simulink model "D53_LKAS_JLU_20200903_0931"  (R2018b)
settings: Solver=ode3  StartTime=0.0  StopTime=10.0  FixedStep=0.01  RelTol=1e-3  EnableMultiTasking=on
model workspace (MAT data in the model file):
  MCOS : class17 (value not decoded)
  MCOS : class17 (value not decoded)
  MCOS : class17 (value not decoded)
  MCOS : class17 (value not decoded)
  MCOS : class17 (value not decoded)
  MCOS : class17 (value not decoded)
  MCOS : class17 (value not decoded)
  MCOS : class17 (value not decoded)
  MCOS : class17 (value not decoded)
  MCOS : class17 (value not decoded)
  MCOS : class17 (value not decoded)
  MCOS : class17 (value not decoded)
  MCOS : class17 (value not decoded)
  MCOS : class17 (value not decoded)
  MCOS : class17 (value not decoded)
  MCOS : class17 (value not decoded)
  MCOS : class17 (value not decoded)
  MCOS : class17 (value not decoded)
  MCOS : class17 (value not decoded)
  MCOS : class17 (value not decoded)
  MCOS : class17 (value not decoded)
  MCOS : class17 (value not decoded)
  MCOS : class17 (value not decoded)
  MCOS : class17 (value not decoded)
  MCOS : class17 (value not decoded)
  MCOS : class17 (value not decoded)
  MCOS : class17 (value not decoded)
  MCOS : class17 (value not decoded)
  MCOS : class17 (value not decoded)
  MCOS : class17 (value not decoded)
  MCOS : class17 (value not decoded)
  MCOS : class17 (value not decoded)
  MCOS : class17 (value not decoded)
  MCOS : class17 (value not decoded)
  MCOS : class17 (value not decoded)
  MCOS : class17 (value not decoded)
  MCOS : class17 (value not decoded)
  MCOS : class17 (value not decoded)
  MCOS : class17 (value not decoded)
  MCOS : class17 (value not decoded)
  MCOS : class17 (value not decoded)
  MCOS : class17 (value not decoded)
  MCOS : class17 (value not decoded)
  MCOS : class17 (value not decoded)
  MCOS : class17 (value not decoded)
  MCOS : class17 (value not decoded)
  MCOS : class17 (value not decoded)
  MCOS : class17 (value not decoded)
  MCOS : class17 (value not decoded)
  MCOS : class17 (value not decoded)
  MCOS : class17 (value not decoded)
  MCOS : class17 (value not decoded)
  MCOS : class17 (value not decoded)
  MCOS : class17 (value not decoded)
  MCOS : class17 (value not decoded)
  MCOS : class17 (value not decoded)
  MCOS : class17 (value not decoded)
  MCOS : class17 (value not decoded)
  MCOS : class17 (value not decoded)
  MCOS : class17 (value not decoded)
  MCOS : class17 (value not decoded)
  MCOS : class17 (value not decoded)
  MCOS : class17 (value not decoded)
  MCOS : class17 (value not decoded)
  MCOS : class17 (value not decoded)
  MCOS : class17 (value not decoded)
  MCOS : class17 (value not decoded)
  MCOS : class17 (value not decoded)
  MCOS : class17 (value not decoded)
  MCOS : class17 (value not decoded)
  MCOS : class17 (value not decoded)
  MCOS : class17 (value not decoded)
  MCOS : class17 (value not decoded)
  MCOS : class17 (value not decoded)
  MCOS : class17 (value not decoded)
  MCOS : class17 (value not decoded)
  MCOS : class17 (value not decoded)
  MCOS : class17 (value not decoded)
  MCOS : class17 (value not decoded)
  MCOS : class17 (value not decoded)
  MCOS : class17 (value not decoded)
  MCOS : class17 (value not decoded)
  MCOS : class17 (value not decoded)
  MCOS : class17 (value not decoded)
  MCOS : class17 (value not decoded)
  MCOS : class17 (value not decoded)
  MCOS : class17 (value not decoded)
  MCOS : class17 (value not decoded)
  MCOS : class17 (value not decoded)
undefined symbols (not defined in the file): LKA_CarWidth, LKA_SampleTime, LKA_StrRatio_C, LKA_Veh2CamL_C, LKA_Veh2CamW_C, LKA_WhlBaseL_C, LL_CompSWA_C, LL_CrvtPrvwT_C, LL_DesDvt_C, LL_DvtComp_C, LL_DvtPrvwT_C, LL_DvtSpdDet_vDvtSpdMin_C, LL_HdAgExT_C, LL_HdAgPrvwT_C, LL_LAccMax_C, LL_LAccRMax_C, LL_LDW_EarliestWarnLine_C, LL_LDW_LatestWarnLine_C, LL_LDWS_SUPPRESS_HEADING, LL_LFClb_TFC_DiffCtlBalance, LL_LFClb_TFC_DiffCtrlMaxSWA, LL_LFClb_TFC_DiffCtrlRatio, LL_LFClb_TFC_facmGainLutGain1_C, LL_LFClb_TFC_facmGainLutGain2_C, LL_LFClb_TFC_facmIntegRatio, LL_LFClb_TFC_facmKlat_C, LL_LFClb_TFC_FfCtlRatio_C, LL_LFClb_TFC_phiIntegCtlMaxSWA_C, LL_LFClb_TFC_tiKlatPrvwT_C, LL_LFClb_TFC_vGainLutVehSpdLwr_C, LL_LFClb_TFC_vGainLutVehSpdUpr_C, LL_LKA_EarliestWarnLine_C, LL_LKA_LatestWarnLine_C, LL_LKAExPrcs_ExitC0Dvt, LL_LKAExPrcs_ExitC0Swt, LL_LKAExPrcs_tiExitTime1, LL_LKAExPrcs_tiExitTime2, LL_LKAExPrcs_tiExitTime3, LL_LKAS_OUT_OF_CONTROL_LAT_VEL, LL_LKAS_OUT_OF_CONTROL_TTLC, LL_LKASWASyn_M0, LL_LKASWASyn_M1, LL_LKASWASyn_M2, LL_LKASWASyn_M3K, LL_LKASWASyn_SWAaddMax, LL_LKASWASyn_T2, LL_LKASWASyn_tiTrqSwaRtTime, LL_LKASWASyn_tiTrqSwaTime, LL_LKASWASyn_TrqMax, LL_LKASWASyn_TrqSwaAddSwt, LL_LKASWASyn_TrqSwaRateDiff, LL_LSpdCompT_C, LL_lStpLngth_C, LL_MAX_DELAY_EPSSTAR_TIME, LL_MAX_DRIVER_TORQUE_DISABLE, LL_MAX_DRIVER_TORQUE_ENABLE, LL_MAX_LANE_WIDTH_DISABLE, LL_MAX_LANE_WIDTH_ENABLE, LL_MAX_LAT_ACC_DISABLE, LL_MAX_LAT_ACC_ENABLE ... (+30)
libraries: simulink x135, canmsglib x41, dspstat3 x3, simulink_extras x1
(part 3 of 18)

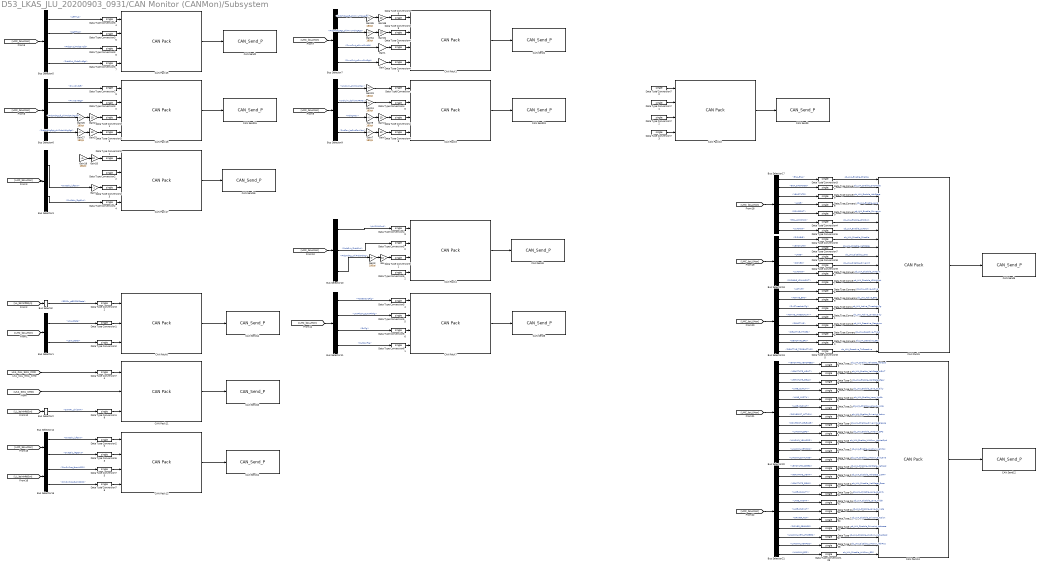
== system D53_LKAS_JLU_20200903_0931/CAN Monitor (CANMon)/Subsystem ==
  Bus Selector : BusSelector  OutputSignals=EPSRx_bsEPSInfo.EPSRx_stEPSCtlState
  Bus Selector1 : BusSelector  OutputSignals=LLStateDetMon.LLState.LKA_State,LLStateDetMon.LLState.LDW_State
  Bus Selector10 : BusSelector  OutputSignals=LKAMon.phiSWACmd,LKAInP_bsLKAInPInfo.signal1.PrdcDvt_bsPrdcDvtInfo.PrdcDvt_lPrdcDvt,LKAInP_bsLKAInPInfo.signal1.PrdcHdAg_bsPrdcHdAgInfo.PrdcHdAg_phiPrdcHdAg
  Bus Selector11 : BusSelector  OutputSignals=LKAMon.LKAPhDet_bsLKAPhDetMon.ToDeactvCFlg,LKAMon.LKAPhDet_bsLKAPhDetMon.LKAPhSM_stLKAPhFlg,LKAMon.LKAPhDet_bsLKAPhDetMon.ExFlg,LKAMon.LKAPhDet_bsLKAPhDetMon.SwtConFlg
  Bus Selector12 : BusSelector  OutputSignals=LLStateDetMon.LLSMConMon.ActvCMon.ACTIVE_THRES.DvtCalc_lLftDvt,LLStateDetMon.LLSMConMon.ActvCMon.ACTIVE_THRES.DvtCalc_lRgtDvt
  Bus Selector15 : BusSelector  OutputSignals=LaneRx_bsLaneInfo.CmrRxPrcs_bsL0Info.CmrRxPrcs_facmL0C0,LaneRx_bsLaneInfo.CmrRxPrcs_bsR0Info.CmrRxPrcs_facmR0C0
  Bus Selector17 : BusSelector  OutputSignals=LLStateDetMon.LLSMConMon.EnaCMon.ENA_ENA,LLStateDetMon.LLSMConMon.EnaCMon.ENA_DACMODE,LLStateDetMon.LLSMConMon.EnaCMon.ENA_VEHSTATE.VEHSTATE,LLStateDetMon.LLSMConMon.EnaCMon.ENA_LANE.LANE,LLStateDetMon.LLSMConMon.EnaCMon.ENA_DRIVERINT.DRIVERINT,LLStateDetMon.LLSMConMon.EnaCMon.ENA_LDWOWN,LLStateDetMon.LLSMConMon.EnaCMon.ENA_LKAOWN.LKAOWN
  Bus Selector18 : BusSelector  OutputSignals=LLStateDetMon.LLSMConMon.DisblCMon.DISABLE,LLStateDetMon.LLSMConMon.DisblCMon.DISABLE_VEHSTATE.VEHSTATE,LLStateDetMon.LLSMConMon.DisblCMon.DISABLE_LANE.LANE,LLStateDetMon.LLSMConMon.DisblCMon.DISABLE_DRIVINT.DRIVER,LLStateDetMon.LLSMConMon.DisblCMon.DISABLE_LKA.LKAOWN,LLStateDetMon.LLSMConMon.DisblCMon.DISABLE_LDWALRMT
  Bus Selector19 : BusSelector  OutputSignals=LLStateDetMon.LLSMConMon.ActvCMon.ACTIVE,LLStateDetMon.LLSMConMon.ActvCMon.ACTIVE_EPS,LLStateDetMon.LLSMConMon.ActvCMon.ACTIVE_THRES.DvtThresActvFlg,LLStateDetMon.LLSMConMon.ActvCMon.ACTIVE_LANEQUALITY,LLStateDetMon.LLSMConMon.DeactvCMon.DEACTIVE,LLStateDetMon.LLSMConMon.DeactvCMon.DEACTIVE_THRES,LLStateDetMon.LLSMConMon.DeactvCMon.DEACTIVE_EPS,LLStateDetMon.LLSMConMon.DeactvCMon.DEACTIVE_TODEACTIVE
  Bus Selector2 : BusSelector  OutputSignals=SWARx_bsSWAInfo.SWARx_phiSWA
  Bus Selector20 : BusSelector  OutputSignals=LLStateDetMon.LLSMConMon.EnaCMon.ENA_VEHSTATE.VEHSTATE_VEHSPEED,LLStateDetMon.LLSMConMon.EnaCMon.ENA_VEHSTATE.VEHSTATE_LIGHT,LLStateDetMon.LLSMConMon.EnaCMon.ENA_VEHSTATE.VEHSTATE_GEAR,LLStateDetMon.LLSMConMon.EnaCMon.ENA_LANE.LANE_QUALITY,LLStateDetMon.LLSMConMon.EnaCMon.ENA_LANE.LANE_WIDTH,LLStateDetMon.LLSMConMon.EnaCMon.ENA_LANE.LANE_CURVAT,LLStateDetMon.LLSMConMon.EnaCMon.ENA_DRIVERINT.DRIVERINT_ACTION,LLStateDetMon.LLSMConMon.EnaCMon.ENA_DRIVERINT.DRIVERINT_RELEASE,LLStateDetMon.LLSMConMon.EnaCMon.ENA_LKAOWN.LKAOWN_EPS,LLStateDetMon.LLSMConMon.EnaCMon.ENA_LKAOWN.LKAOWN_VEHLSPD,LLStateDetMon.LLSMConMon.EnaCMon.ENA_LKAOWN.LKAOWN_VEHPOS,LLStateDetMon.LLSMConMon.EnaCMon.ENA_LKAOWN.LKAOWN_EXITLANE
  Bus Selector21 : BusSelector  OutputSignals=LLStateDetMon.LLSMConMon.DisblCMon.DISABLE_VEHSTATE.VEHSTATE_SPEED,LLStateDetMon.LLSMConMon.DisblCMon.DISABLE_VEHSTATE.VEHSTATE_LIGHT,LLStateDetMon.LLSMConMon.DisblCMon.DISABLE_VEHSTATE.VEHSTATE_GEAR,LLStateDetMon.LLSMConMon.DisblCMon.DISABLE_LANE.LANE_QUALITY,LLStateDetMon.LLSMConMon.DisblCMon.DISABLE_LANE.LANE_WIDTH,LLStateDetMon.LLSMConMon.DisblCMon.DISABLE_LANE.LANE_CURVAT,LLStateDetMon.LLSMConMon.DisblCMon.DISABLE_DRIVINT.DRIVER_ACT,LLStateDetMon.LLSMConMon.DisblCMon.DISABLE_DRIVINT.DRIVER_RELEASE,LLStateDetMon.LLSMConMon.DisblCMon.DISABLE_LKA.LKAOWN_VEHLATSPEED,LLStateDetMon.LLSMConMon.DisblCMon.DISABLE_LKA.LKAOWN_VEHPOS,LLStateDetMon.LLSMConMon.DisblCMon.DISABLE_LKA.LKAOWN_EPS
  Bus Selector3 : BusSelector  OutputSignals=LLStateDetMon.LLSMConMon.ActvCMon.ACTIVE_THRES.DvtCalc_lLftDvt,LLStateDetMon.LLSMConMon.ActvCMon.ACTIVE_THRES.DvtCalc_lRgtDvt
  Bus Selector5 : BusSelector  OutputSignals=LLStateDetMon.LLSMConMon.TTLCMon.LftTTLC,LLStateDetMon.LLSMConMon.TTLCMon.RgtTTLC,LKAInP_bsLKAInPInfo.signal1.PrdcDvt_bsPrdcDvtInfo.PrdcDvt_lPrdcDvtLft,LKAInP_bsLKAInPInfo.signal1.PrdcDvt_bsPrdcDvtInfo.PrdcDvt_lPrdcDvtRgt
  Bus Selector6 : BusSelector  OutputSignals=LKAInP_bsLKAInPMon.PrdcDvtCal_bsPrdcDvtCalMon.DvtLftMon.PrvwDvtLft,LKAInP_bsLKAInPMon.PrdcDvtCal_bsPrdcDvtCalMon.DvtRgtMon.PrvwDvtRgt,LKAInP_bsLKAInPInfo.signal1.PrdcHdAg_bsPrdcHdAgInfo.PrdcHdAgLft_phiPrdcHdAgLft,LKAInP_bsLKAInPInfo.signal1.PrdcHdAg_bsPrdcHdAgInfo.PrdcHdAgRgt_phiPrdcHdAgRgt
  Bus Selector7 : BusSelector  OutputSignals=LKAInP_bsLKAInPMon.PrdcHdAg_bsPrdcHdAgMon.PrdcHdAgLft_phiPrvwHdAgLft,LKAInP_bsLKAInPMon.PrdcHdAg_bsPrdcHdAgMon.PrdcHdAgRgt_phiPrvwHdAgRgt,LKAInP_bsLKAInPInfo.signal1.PrvwCrvt_bsPrvwCrvtInfo.PrvwCrvt_crPrvwCrvtLft,LKAInP_bsLKAInPInfo.signal1.PrvwCrvt_bsPrvwCrvtInfo.PrvwCrvt_crPrvwCrvtRgt
  Bus Selector9 : BusSelector  OutputSignals=LKAInP_bsLKAInPInfo.UndrLim_phiSWAMax,LKAInP_bsLKAInPInfo.UndrLim_dphiSWARMax,LKAMon.LKAPhDet_bsLKAPhDetMon.HdAgMax,LKAMon.LKAPhDet_bsLKAPhDetMon.SwtCon_bsSwtConMon
  CAN Pack1 : canmsglib/CAN Pack  CANdbFile=C:\Users\Administrator\Desktop\data_collect.dbc  MsgList=(none)  MsgName=c1deg  MsgIDType=Standard (11-bit identifier)  MsgIdentifier=2018  MsgLength=8  SignalInfo=PrdcHdAgLft_phiPrvwHdAgLft$8$16$2$1$1$0$0.01$0$-320$320$#PrdcHdAgRgt_phiPrvwHdAgRgt$24$16$2$1$1$0$0.01$0$-320$320$#PrvwCrvt_crPrvwCrvLft$40$16$2$1$1$0$0.01$0$-320$320$#PrvwCrvt_crPrvwCrvRgt$56$16$2$1$1$0$0.01$0$-320$320$#  NSignals=4  StartBits=str2num('[int32(8);int32(24);int32(40);int32(56)]')  SignalSizes=str2num('[int32(16);int32(16);int32(16);int32(16)]')  ByteOrders=str2num('[int32(2);int32(2);int32(2);int32(2)]')  DataTypes=str2num('[int32(1);int32(1);int32(1);int32(1)]')  MultiplexTypes=str2num('[int32(1);int32(1);int32(1);int32(1)]')  MultiplexValues=str2num('[double(0);double(0);double(0);double(0)]')  Factors=str2num('[double(0.01);double(0.01);double(0.01);double(0.01)]')  Offsets=str2num('[double(0);double(0);double(0);double(0)]')  Minimums=str2num('[double(-320);double(-320);double(-320);double(-320)]')  Maximums=str2num('[double(320);double(320);double(320);double(320)]')  Remote=off  ApplyMinMax=off  BusOutput=off
      settings: SourceProductName=Simulink Real-Time  SourceProductBaseCode=XP  DataFormat=manually specified signals
  CAN Pack10 : canmsglib/CAN Pack  CANdbFile=C:\Users\Administrator\Desktop\data_collect.dbc  MsgList=(none)  MsgName=c1deg1  MsgIDType=Standard (11-bit identifier)  MsgIdentifier=40  MsgLength=8  SignalInfo=signal00001$8$16$2$1$1$0$0.01$0$-320$320$#signal00002$24$16$2$1$1$0$0.01$0$-320$320$#signal00003$40$16$2$1$1$0$1.000000e-002$0$-320$320$#signal00004$56$16$2$1$1$0$1.000000e-002$0$-320$320$#  NSignals=4  StartBits=str2num('[int32(8);int32(24);int32(40);int32(56)]')  SignalSizes=str2num('[int32(16);int32(16);int32(16);int32(16)]')  ByteOrders=str2num('[int32(2);int32(2);int32(2);int32(2)]')  DataTypes=str2num('[int32(1);int32(1);int32(1);int32(1)]')  MultiplexTypes=str2num('[int32(1);int32(1);int32(1);int32(1)]')  MultiplexValues=str2num('[double(0);double(0);double(0);double(0)]')  Factors=str2num('[double(0.01);double(0.01);double(1.000000e-002);double(1.000000e-002)]')  Offsets=str2num('[double(0);double(0);double(0);double(0)]')  Minimums=str2num('[double(-320);double(-320);double(-320);double(-320)]')  Maximums=str2num('[double(320);double(320);double(320);double(320)]')  Remote=off  ApplyMinMax=off  BusOutput=off
      settings: SourceProductName=Simulink Real-Time  SourceProductBaseCode=XP  DataFormat=manually specified signals
  CAN Pack11 : canmsglib/CAN Pack  CANdbFile=F:\LD\1_simulink\GateWay_20180716\dbc\camera_data_in.dbc  MsgList=(none)  MsgName=LKAFlag  MsgIDType=Standard (11-bit identifier)  MsgIdentifier=2025  MsgLength=8  SignalInfo=LKA_CAL_SWA_CMD$8$16$2$1$1$0$0.1$0$-Inf$Inf$#SWA_CMD$24$16$2$1$1$0$0.1$0$-Inf$Inf$#SWA_Signal$40$16$2$1$1$0$0.1$0$-Inf$Inf$#  NSignals=3  StartBits=str2num('[int32(8);int32(24);int32(40)]')  SignalSizes=str2num('[int32(16);int32(16);int32(16)]')  ByteOrders=str2num('[int32(2);int32(2);int32(2)]')  DataTypes=str2num('[int32(1);int32(1);int32(1)]')  MultiplexTypes=str2num('[int32(1);int32(1);int32(1)]')  MultiplexValues=str2num('[double(0);double(0);double(0)]')  Factors=str2num('[double(0.1);double(0.1);double(0.1)]')  Offsets=str2num('[double(0);double(0);double(0)]')  Minimums=str2num('[double(-Inf);double(-Inf);double(-Inf)]')  Maximums=str2num('[double(Inf);double(Inf);double(Inf)]')  Remote=off  ApplyMinMax=off  BusOutput=off
      settings: SourceProductName=Simulink Real-Time  SourceProductBaseCode=XP  DataFormat=manually specified signals
  CAN Pack12 : canmsglib/CAN Pack  CANdbFile=F:\LD\1_simulink\GateWay_20180716\dbc\camera_data_in.dbc  MsgList=(none)  MsgName=LKAFlag  MsgIDType=Standard (11-bit identifier)  MsgIdentifier=2026  MsgLength=8  SignalInfo=LFT_DVT$8$16$2$1$1$0$0.01$0$-Inf$Inf$#RGT_DVT$24$16$2$1$1$0$0.01$0$-Inf$Inf$#L0$40$16$2$1$1$0$0.01$0$-Inf$Inf$#R0$56$16$2$1$1$0$0.01$0$-Inf$Inf$#  NSignals=4  StartBits=str2num('[int32(8);int32(24);int32(40);int32(56)]')  SignalSizes=str2num('[int32(16);int32(16);int32(16);int32(16)]')  ByteOrders=str2num('[int32(2);int32(2);int32(2);int32(2)]')  DataTypes=str2num('[int32(1);int32(1);int32(1);int32(1)]')  MultiplexTypes=str2num('[int32(1);int32(1);int32(1);int32(1)]')  MultiplexValues=str2num('[double(0);double(0);double(0);double(0)]')  Factors=str2num('[double(0.01);double(0.01);double(0.01);double(0.01)]')  Offsets=str2num('[double(0);double(0);double(0);double(0)]')  Minimums=str2num('[double(-Inf);double(-Inf);double(-Inf);double(-Inf)]')  Maximums=str2num('[double(Inf);double(Inf);double(Inf);double(Inf)]')  Remote=off  ApplyMinMax=off  BusOutput=off
      settings: SourceProductName=Simulink Real-Time  SourceProductBaseCode=XP  DataFormat=manually specified signals
  CAN Pack13 : canmsglib/CAN Pack  CANdbFile=C:\Users\Administrator\Desktop\data_collect.dbc  MsgList=(none)  MsgName=c1deg1  MsgIDType=Standard (11-bit identifier)  MsgIdentifier=99  MsgLength=8  SignalInfo=ob_LKA_Enable_VehState_VehSpd$0$2$1$2$1$0$1$0$0$3$#ob_LKA_Enable_VehState_LIGHT$2$2$1$2$1$0$1$0$0$3$#ob_LKA_Enable_VehState_Gear$4$2$1$2$1$0$1$0$0$3$#ob_LKA_Enable_Lane_Quality$6$2$1$2$1$0$1$0$0$3$#ob_LKA_Enable_Lane_Width$8$2$1$2$1$0$1$0$0$3$#ob_LKA_Enable_Lane_Curvate$10$2$1$2$1$0$1$0$0$3$#ob_LKA_Enable_DriverInt_Action$12$2$1$2$1$0$1$0$0$3$#ob_LKA_Enable_DriverInt_Release$14$2$1$2$1$0$1$0$0$3$#ob_LKA_Enable_LKAOwn_EPS$16$2$1$2$1$0$1$0$0$3$#ob_LKA_Enable_LKAOwn_VehLatSpd$18$2$1$2$1$0$1$0$0$3$#ob_LKA_Enable_LKAOwn_VehPos$20$2$1$2$1$0$1$0$0$3$#ob_LKA_Enable_LKAOwn_ExitLane$22$2$1$2$1$0$1$0$0$3$#ob_LKA_Disable_VehState_VehSpd$24$2$1$2$1$0$1$0$0$3$#ob_LKA_Disable_VehState_LIGHT$26$2$1$1$1$0$1$0$-Inf$Inf$#ob_LKA_Disable_VehState_Gear$28$2$1$1$1$0$1$0$-Inf$Inf$#ob_LKA_Disable_Lane_Quality$30$2$1$1$1$0$1$0$-Inf$Inf$#ob_LKA_Disable_Lane_Width$32$2$1$1$1$0$1$0$-Inf$Inf$#ob_LKA_Disable_Lane_Curvate$34$2$1$1$1$0$1$0$-Inf$Inf$#ob_LKA_Disable_DriverInt_Action$36$2$1$1$1$0$1$0$-Inf$Inf$#ob_LKA_Disable_DriverInt_Release$38$2$1$1$1$0$1$0$-Inf$Inf$#ob_LKA_Disable_LKAOwn_VehLatSpd$40$2$1$1$1$0$1$0$-Inf$Inf$#ob_LKA_Disable_LKAOwn_VehPos$42$2$1$1$1$0$1$0$-Inf$Inf$#ob_LKA_Disable_LKAOwn_EPS$44$2$1$1$1$0$1$0$-Inf$Inf$#  NSignals=23  StartBits=str2num('[int32(0);int32(2);int32(4);int32(6);int32(8);int32(10);int32(12);int32(14);int32(16);int32(18);int32(20);int32(22);int32(24);int32(26);int32(28);int32(30);int32(32);int32(34);int32(36);int32(38);int32(40);int32(42);int32(44)]')  SignalSizes=str2num('[int32(2);int32(2);int32(2);int32(2);int32(2);int32(2);int32(2);int32(2);int32(2);int32(2);int32(2);int32(2);int32(2);int32(2);int32(2);int32(2);int32(2);int32(2);int32(2);int32(2);int32(2);int32(2);int32(2)]')  ByteOrders=str2num('[int32(1);int32(1);int32(1);int32(1);int32(1);int32(1);int32(1);int32(1);int32(1);int32(1);int32(1);int32(1);int32(1);int32(1);int32(1);int32(1);int32(1);int32(1);int32(1);int32(1);int32(1);int32(1);int32(1)]')  DataTypes=str2num('[int32(2);int32(2);int32(2);int32(2);int32(2);int32(2);int32(2);int32(2);int32(2);int32(2);int32(2);int32(2);int32(2);int32(1);int32(1);int32(1);int32(1);int32(1);int32(1);int32(1);int32(1);int32(1);int32(1)]')  MultiplexTypes=str2num('[int32(1);int32(1);int32(1);int32(1);int32(1);int32(1);int32(1);int32(1);int32(1);int32(1);int32(1);int32(1);int32(1);int32(1);int32(1);int32(1);int32(1);int32(1);int32(1);int32(1);int32(1);int32(1);int32(1)]')  MultiplexValues=str2num('[double(0);double(0);double(0);double(0);double(0);double(0);double(0);double(0);double(0);double(0);double(0);double(0);double(0);double(0);double(0);double(0);double(0);double(0);double(0);double(0);double(0);double(0);double(0)]')  Factors=str2num('[double(1);double(1);double(1);double(1);double(1);double(1);double(1);double(1);double(1);double(1);double(1);double(1);double(1);double(1);double(1);double(1);double(1);double(1);double(1);double(1);double(1);double(1);double(1)]')  Offsets=str2num('[double(0);double(0);double(0);double(0);double(0);double(0);double(0);double(0);double(0);double(0);double(0);double(0);double(0);double(0);double(0);double(0);double(0);double(0);double(0);double(0);double(0);double(0);double(0)]')  Minimums=str2num('[double(0);double(0);double(0);double(0);double(0);double(0);double(0);double(0);double(0);double(0);double(0);double(0);double(0);double(-Inf);double(-Inf);double(-Inf);double(-Inf);double(-Inf);double(-Inf);double(-Inf);double(-Inf);double(-Inf);double(-Inf)]')  Maximums=str2num('[double(3);double(3);double(3);double(3);double(3);double(3);double(3);double(3);double(3);double(3);double(3);double(3);double(3);double(Inf);double(Inf);double(Inf);double(Inf);double(Inf);double(Inf);double(Inf);double(Inf);double(Inf);double(Inf)]')  Remote=off  ApplyMinMax=off  BusOutput=off
      settings: SourceProductName=Simulink Real-Time  SourceProductBaseCode=XP  DataFormat=manually specified signals
  CAN Pack15 : canmsglib/CAN Pack  CANdbFile=C:\Users\Administrator\Desktop\data_collect.dbc  MsgList=(none)  MsgName=c1deg  MsgIDType=Standard (11-bit identifier)  MsgIdentifier=27  MsgLength=8  SignalInfo=LFT_TTLC$8$16$2$1$1$0$0.01$0$-320$320$#RGT_TTLC$24$16$2$1$1$0$0.01$0$-320$320$#PrdcDvt_IPrdcDvtLft$40$16$2$1$1$0$1.000000e-002$0$-320$320$#PrdcDvt_IPrdcDvtRgt$56$16$2$1$1$0$1.000000e-002$0$-320$320$#  NSignals=4  StartBits=str2num('[int32(8);int32(24);int32(40);int32(56)]')  SignalSizes=str2num('[int32(16);int32(16);int32(16);int32(16)]')  ByteOrders=str2num('[int32(2);int32(2);int32(2);int32(2)]')  DataTypes=str2num('[int32(1);int32(1);int32(1);int32(1)]')  MultiplexTypes=str2num('[int32(1);int32(1);int32(1);int32(1)]')  MultiplexValues=str2num('[double(0);double(0);double(0);double(0)]')  Factors=str2num('[double(0.01);double(0.01);double(1.000000e-002);double(1.000000e-002)]')  Offsets=str2num('[double(0);double(0);double(0);double(0)]')  Minimums=str2num('[double(-320);double(-320);double(-320);double(-320)]')  Maximums=str2num('[double(320);double(320);double(320);double(320)]')  Remote=off  ApplyMinMax=off  BusOutput=off
      settings: SourceProductName=Simulink Real-Time  SourceProductBaseCode=XP  DataFormat=manually specified signals
  CAN Pack16 : canmsglib/CAN Pack  CANdbFile=C:\Users\Administrator\Desktop\data_collect.dbc  MsgList=(none)  MsgName=c1deg  MsgIDType=Standard (11-bit identifier)  MsgIdentifier=28  MsgLength=8  SignalInfo=PrvwDvtLft$8$16$2$1$1$0$0.01$0$-320$320$#PrvwDvtRgt$24$16$2$1$1$0$0.01$0$-320$320$#PrdcHdAgLft_phiPrdcHdAgLft$40$16$2$1$1$0$1.000000e-002$0$-320$320$#PrdcHdAgRgt_phiPrdcHdAgRgt$56$16$2$1$1$0$1.000000e-002$0$-320$320$#  NSignals=4  StartBits=str2num('[int32(8);int32(24);int32(40);int32(56)]')  SignalSizes=str2num('[int32(16);int32(16);int32(16);int32(16)]')  ByteOrders=str2num('[int32(2);int32(2);int32(2);int32(2)]')  DataTypes=str2num('[int32(1);int32(1);int32(1);int32(1)]')  MultiplexTypes=str2num('[int32(1);int32(1);int32(1);int32(1)]')  MultiplexValues=str2num('[double(0);double(0);double(0);double(0)]')  Factors=str2num('[double(0.01);double(0.01);double(1.000000e-002);double(1.000000e-002)]')  Offsets=str2num('[double(0);double(0);double(0);double(0)]')  Minimums=str2num('[double(-320);double(-320);double(-320);double(-320)]')  Maximums=str2num('[double(320);double(320);double(320);double(320)]')  Remote=off  ApplyMinMax=off  BusOutput=off
      settings: SourceProductName=Simulink Real-Time  SourceProductBaseCode=XP  DataFormat=manually specified signals
  CAN Pack17 : canmsglib/CAN Pack  CANdbFile=C:\Users\Administrator\Desktop\data_collect.dbc  MsgList=(none)  MsgName=c1deg  MsgIDType=Standard (11-bit identifier)  MsgIdentifier=29  MsgLength=8  SignalInfo=LKATG_phiDesHdAg$8$16$2$1$1$0$0.01$0$-320$320$#LKATG_IDesDvt$24$16$2$1$1$0$0.01$0$-320$320$#DvtCalc_ILftDvt$40$16$2$1$1$0$0.01$0$-320$320$#DvtCalc_IRgtDvt$56$16$2$1$1$0$0.01$0$-320$320$#  NSignals=4  StartBits=str2num('[int32(8);int32(24);int32(40);int32(56)]')  SignalSizes=str2num('[int32(16);int32(16);int32(16);int32(16)]')  ByteOrders=str2num('[int32(2);int32(2);int32(2);int32(2)]')  DataTypes=str2num('[int32(1);int32(1);int32(1);int32(1)]')  MultiplexTypes=str2num('[int32(1);int32(1);int32(1);int32(1)]')  MultiplexValues=str2num('[double(0);double(0);double(0);double(0)]')  Factors=str2num('[double(0.01);double(0.01);double(0.01);double(0.01)]')  Offsets=str2num('[double(0);double(0);double(0);double(0)]')  Minimums=str2num('[double(-320);double(-320);double(-320);double(-320)]')  Maximums=str2num('[double(320);double(320);double(320);double(320)]')  Remote=off  ApplyMinMax=off  BusOutput=off
      settings: SourceProductName=Simulink Real-Time  SourceProductBaseCode=XP  DataFormat=manually specified signals
  CAN Pack3 : canmsglib/CAN Pack  CANdbFile=C:\Users\Administrator\Desktop\data_collect.dbc  MsgList=(none)  MsgName=c1deg  MsgIDType=Standard (11-bit identifier)  MsgIdentifier=2019  MsgLength=8  SignalInfo=L0_C1_deg$8$16$2$1$1$0$0.01$0$-320$320$#R0_C1_deg$24$16$2$1$1$0$0.01$0$-320$320$#L0_C0_cal$40$16$2$1$1$0$0.01$0$-320$320$#R0_C0_cal$56$16$2$1$1$0$0.01$0$-320$320$#  NSignals=4  StartBits=str2num('[int32(8);int32(24);int32(40);int32(56)]')  SignalSizes=str2num('[int32(16);int32(16);int32(16);int32(16)]')  ByteOrders=str2num('[int32(2);int32(2);int32(2);int32(2)]')  DataTypes=str2num('[int32(1);int32(1);int32(1);int32(1)]')  MultiplexTypes=str2num('[int32(1);int32(1);int32(1);int32(1)]')  MultiplexValues=str2num('[double(0);double(0);double(0);double(0)]')  Factors=str2num('[double(0.01);double(0.01);double(0.01);double(0.01)]')  Offsets=str2num('[double(0);double(0);double(0);double(0)]')  Minimums=str2num('[double(-320);double(-320);double(-320);double(-320)]')  Maximums=str2num('[double(320);double(320);double(320);double(320)]')  Remote=off  ApplyMinMax=off  BusOutput=off
      settings: SourceProductName=Simulink Real-Time  SourceProductBaseCode=XP  DataFormat=manually specified signals
  CAN Pack4 : canmsglib/CAN Pack  CANdbFile=C:\Users\Administrator\Desktop\data_collect.dbc  MsgList=(none)  MsgName=c1deg1  MsgIDType=Standard (11-bit identifier)  MsgIdentifier=33  MsgLength=8  SignalInfo=signal00001$8$16$2$1$1$0$0.01$0$-320$320$#signal00002$24$16$2$1$1$0$0.01$0$-320$320$#signal00003$40$16$2$1$1$0$1.000000e-002$0$-320$320$#signal00004$56$16$2$1$1$0$1.000000e-002$0$-320$320$#  NSignals=4  StartBits=str2num('[int32(8);int32(24);int32(40);int32(56)]')  SignalSizes=str2num('[int32(16);int32(16);int32(16);int32(16)]')  ByteOrders=str2num('[int32(2);int32(2);int32(2);int32(2)]')  DataTypes=str2num('[int32(1);int32(1);int32(1);int32(1)]')  MultiplexTypes=str2num('[int32(1);int32(1);int32(1);int32(1)]')  MultiplexValues=str2num('[double(0);double(0);double(0);double(0)]')  Factors=str2num('[double(0.01);double(0.01);double(1.000000e-002);double(1.000000e-002)]')  Offsets=str2num('[double(0);double(0);double(0);double(0)]')  Minimums=str2num('[double(-320);double(-320);double(-320);double(-320)]')  Maximums=str2num('[double(320);double(320);double(320);double(320)]')  Remote=off  ApplyMinMax=off  BusOutput=off
      settings: SourceProductName=Simulink Real-Time  SourceProductBaseCode=XP  DataFormat=manually specified signals
  CAN Pack5 : canmsglib/CAN Pack  CANdbFile=C:\Users\Administrator\Desktop\data_collect.dbc  MsgList=(none)  MsgName=c1deg1  MsgIDType=Standard (11-bit identifier)  MsgIdentifier=98  MsgLength=8  SignalInfo=ob_LKA_Enable_Enable$0$2$1$2$1$0$1$0$0$3$#ob_LKA_Enable_DACMode$2$2$1$2$1$0$1$0$0$3$#ob_LKA_Enable_VehState$4$2$1$2$1$0$1$0$0$3$#ob_LKA_Enable_Lane$6$2$1$2$1$0$1$0$0$3$#ob_LKA_Enable_DriverInt$8$2$1$2$1$0$1$0$0$3$#ob_LKA_Enable_LDWOwn$10$2$1$2$1$0$1$0$0$3$#ob_LKA_Enable_LKAOwn$12$2$1$2$1$0$1$0$0$3$#ob_LKA_Disable_Disable$14$2$1$2$1$0$1$0$0$3$#ob_LKA_Disable_VehState$16$2$1$2$1$0$1$0$0$3$#ob_LKA_Disable_Lane$18$2$1$2$1$0$1$0$0$3$#ob_LKA_Disable_DriverInt$20$2$1$2$1$0$1$0$0$3$#ob_LKA_Disable_LKAOwn$22$2$1$2$1$0$1$0$0$3$#ob_LKA_Disable_LDWAlrmt$24$2$1$2$1$0$1$0$0$3$#ob_LKA_Active_Active$26$2$1$1$1$0$1$0$-Inf$Inf$#ob_LKA_Active_EPS$28$2$1$1$1$0$1$0$-Inf$Inf$#ob_LKA_Active_ThresActvFlg$30$2$1$1$1$0$1$0$-Inf$Inf$#ob_LKA_Active_LaneQuality$32$2$1$1$1$0$1$0$-Inf$Inf$#ob_LKA_Deactive_Deactive$34$2$1$1$1$0$1$0$-Inf$Inf$#ob_LKA_Deactive_Thres$36$2$1$1$1$0$1$0$-Inf$Inf$#ob_LKA_Deactive_EPS$38$2$1$1$1$0$1$0$-Inf$Inf$#ob_LKA_Deactive_ToDeactive$40$2$1$1$1$0$1$0$-Inf$Inf$#  NSignals=21  StartBits=str2num('[int32(0);int32(2);int32(4);int32(6);int32(8);int32(10);int32(12);int32(14);int32(16);int32(18);int32(20);int32(22);int32(24);int32(26);int32(28);int32(30);int32(32);int32(34);int32(36);int32(38);int32(40)]')  SignalSizes=str2num('[int32(2);int32(2);int32(2);int32(2);int32(2);int32(2);int32(2);int32(2);int32(2);int32(2);int32(2);int32(2);int32(2);int32(2);int32(2);int32(2);int32(2);int32(2);int32(2);int32(2);int32(2)]')  ByteOrders=str2num('[int32(1);int32(1);int32(1);int32(1);int32(1);int32(1);int32(1);int32(1);int32(1);int32(1);int32(1);int32(1);int32(1);int32(1);int32(1);int32(1);int32(1);int32(1);int32(1);int32(1);int32(1)]')  DataTypes=str2num('[int32(2);int32(2);int32(2);int32(2);int32(2);int32(2);int32(2);int32(2);int32(2);int32(2);int32(2);int32(2);int32(2);int32(1);int32(1);int32(1);int32(1);int32(1);int32(1);int32(1);int32(1)]')  MultiplexTypes=str2num('[int32(1);int32(1);int32(1);int32(1);int32(1);int32(1);int32(1);int32(1);int32(1);int32(1);int32(1);int32(1);int32(1);int32(1);int32(1);int32(1);int32(1);int32(1);int32(1);int32(1);int32(1)]')  MultiplexValues=str2num('[double(0);double(0);double(0);double(0);double(0);double(0);double(0);double(0);double(0);double(0);double(0);double(0);double(0);double(0);double(0);double(0);double(0);double(0);double(0);double(0);double(0)]')  Factors=str2num('[double(1);double(1);double(1);double(1);double(1);double(1);double(1);double(1);double(1);double(1);double(1);double(1);double(1);double(1);double(1);double(1);double(1);double(1);double(1);double(1);double(1)]')  Offsets=str2num('[double(0);double(0);double(0);double(0);double(0);double(0);double(0);double(0);double(0);double(0);double(0);double(0);double(0);double(0);double(0);double(0);double(0);double(0);double(0);double(0);double(0)]')  Minimums=str2num('[double(0);double(0);double(0);double(0);double(0);double(0);double(0);double(0);double(0);double(0);double(0);double(0);double(0);double(-Inf);double(-Inf);double(-Inf);double(-Inf);double(-Inf);double(-Inf);double(-Inf);double(-Inf)]')  Maximums=str2num('[double(3);double(3);double(3);double(3);double(3);double(3);double(3);double(3);double(3);double(3);double(3);double(3);double(3);double(Inf);double(Inf);double(Inf);double(Inf);double(Inf);double(Inf);double(Inf);double(Inf)]')  Remote=off  ApplyMinMax=off  BusOutput=off
      settings: SourceProductName=Simulink Real-Time  SourceProductBaseCode=XP  DataFormat=manually specified signals
  CAN Pack6 : canmsglib/CAN Pack  CANdbFile=F:\LD\1_simulink\GateWay_20180716\dbc\camera_data_in.dbc  MsgList=(none)  MsgName=LKAFlag  MsgIDType=Standard (11-bit identifier)  MsgIdentifier=2024  MsgLength=8  SignalInfo=EPS_Status$0$2$1$2$1$0$1$0$0$4$#LKA_Status$2$4$1$2$1$0$1$0$0$16$#LDW_Status$6$4$1$2$1$0$1$0$0$16$#  NSignals=3  StartBits=str2num('[int32(0);int32(2);int32(6)]')  SignalSizes=str2num('[int32(2);int32(4);int32(4)]')  ByteOrders=str2num('[int32(1);int32(1);int32(1)]')  DataTypes=str2num('[int32(2);int32(2);int32(2)]')  MultiplexTypes=str2num('[int32(1);int32(1);int32(1)]')  MultiplexValues=str2num('[double(0);double(0);double(0)]')  Factors=str2num('[double(1);double(1);double(1)]')  Offsets=str2num('[double(0);double(0);double(0)]')  Minimums=str2num('[double(0);double(0);double(0)]')  Maximums=str2num('[double(4);double(16);double(16)]')  Remote=off  ApplyMinMax=off  BusOutput=off
      settings: SourceProductName=Simulink Real-Time  SourceProductBaseCode=XP  DataFormat=manually specified signals
  CAN Pack7 : canmsglib/CAN Pack  CANdbFile=C:\Users\Administrator\Desktop\data_collect.dbc  MsgList=(none)  MsgName=c1deg1  MsgIDType=Standard (11-bit identifier)  MsgIdentifier=35  MsgLength=8  SignalInfo=ToDeactvCflg$8$16$2$1$1$0$0.01$0$-320$320$#LKAPhSM_stLKAPhFlg$24$16$2$1$1$0$0.01$0$-320$320$#ExFlg$40$16$2$1$1$0$0.01$0$-320$320$#SwtConFlg$56$16$2$1$1$0$0.01$0$-320$320$#  NSignals=4  StartBits=str2num('[int32(8);int32(24);int32(40);int32(56)]')  SignalSizes=str2num('[int32(16);int32(16);int32(16);int32(16)]')  ByteOrders=str2num('[int32(2);int32(2);int32(2);int32(2)]')  DataTypes=str2num('[int32(1);int32(1);int32(1);int32(1)]')  MultiplexTypes=str2num('[int32(1);int32(1);int32(1);int32(1)]')  MultiplexValues=str2num('[double(0);double(0);double(0);double(0)]')  Factors=str2num('[double(0.01);double(0.01);double(0.01);double(0.01)]')  Offsets=str2num('[double(0);double(0);double(0);double(0)]')  Minimums=str2num('[double(-320);double(-320);double(-320);double(-320)]')  Maximums=str2num('[double(320);double(320);double(320);double(320)]')  Remote=off  ApplyMinMax=off  BusOutput=off
      settings: SourceProductName=Simulink Real-Time  SourceProductBaseCode=XP  DataFormat=manually specified signals
  CAN Send1 : S-Function  FunctionName=CAN_Send_P  Parameters=uint8(CAN_Port-1),uint8(CAN_Priority-1),uint8(S_overflow_flag),uint8(S_timestamp),double(sampletime)  SFunctionDeploymentMode=off  EnableBusSupport=off  mask{CAN_Port=CAN_0, CAN_Priority=3, S_overflow_flag=off, S_timestamp=off, sampletime=0.01}
      mask prompts: CAN_Port "CAN Port:"; CAN_Priority "Priority:"; S_overflow_flag "Send overflow flag"; S_timestamp "Send time stamp"
      mask init:
      | maskdisplay = cansendicon(CAN_Port,CAN_Priority,S_overflow_flag,S_timestamp);
      | set_param(gcb, 'MaskDisplay', maskdisplay);
      mask TypeOptions CAN_Port: CAN_0 | CAN_1 | CAN_2 | CAN_3
      mask TypeOptions CAN_Priority: 0 | 1 | 2 | 3 | 4 | 5 | 6 | 7
      mask Display: color('blue');text(0.98,0.9,'MPC5675K','horizontalAlignment','right');color('black');text(0.5,0.6,'FlexCAN_0 Send','horizontalAlignment','center');text(0.5,0.35,'Priority:3','horizontalAlignment','center');port_label('input',1,'CAN_Msg');
  CAN Send10 : S-Function  FunctionName=CAN_Send_P  Parameters=uint8(CAN_Port-1),uint8(CAN_Priority-1),uint8(S_overflow_flag),uint8(S_timestamp),double(sampletime)  SFunctionDeploymentMode=off  EnableBusSupport=off  mask{CAN_Port=CAN_0, CAN_Priority=3, S_overflow_flag=off, S_timestamp=off, sampletime=0.01}
      mask prompts: CAN_Port "CAN Port:"; CAN_Priority "Priority:"; S_overflow_flag "Send overflow flag"; S_timestamp "Send time stamp"
      mask init:
      | maskdisplay = cansendicon(CAN_Port,CAN_Priority,S_overflow_flag,S_timestamp);
      | set_param(gcb, 'MaskDisplay', maskdisplay);
      mask TypeOptions CAN_Port: CAN_0 | CAN_1 | CAN_2 | CAN_3
      mask TypeOptions CAN_Priority: 0 | 1 | 2 | 3 | 4 | 5 | 6 | 7
      mask Display: color('blue');text(0.98,0.9,'MPC5675K','horizontalAlignment','right');color('black');text(0.5,0.6,'FlexCAN_0 Send','horizontalAlignment','center');text(0.5,0.35,'Priority:3','horizontalAlignment','center');port_label('input',1,'CAN_Msg');
  CAN Send11 : S-Function  FunctionName=CAN_Send_P  Parameters=uint8(CAN_Port-1),uint8(CAN_Priority-1),uint8(S_overflow_flag),uint8(S_timestamp),double(sampletime)  SFunctionDeploymentMode=off  EnableBusSupport=off  mask{CAN_Port=CAN_0, CAN_Priority=3, S_overflow_flag=off, S_timestamp=off, sampletime=0.01}
      mask prompts: CAN_Port "CAN Port:"; CAN_Priority "Priority:"; S_overflow_flag "Send overflow flag"; S_timestamp "Send time stamp"
      mask init:
      | maskdisplay = cansendicon(CAN_Port,CAN_Priority,S_overflow_flag,S_timestamp);
      | set_param(gcb, 'MaskDisplay', maskdisplay);
      mask TypeOptions CAN_Port: CAN_0 | CAN_1 | CAN_2 | CAN_3
      mask TypeOptions CAN_Priority: 0 | 1 | 2 | 3 | 4 | 5 | 6 | 7
      mask Display: color('blue');text(0.98,0.9,'MPC5675K','horizontalAlignment','right');color('black');text(0.5,0.6,'FlexCAN_0 Send','horizontalAlignment','center');text(0.5,0.35,'Priority:3','horizontalAlignment','center');port_label('input',1,'CAN_Msg');
  CAN Send12 : S-Function  FunctionName=CAN_Send_P  Parameters=uint8(CAN_Port-1),uint8(CAN_Priority-1),uint8(S_overflow_flag),uint8(S_timestamp),double(sampletime)  SFunctionDeploymentMode=off  EnableBusSupport=off  mask{CAN_Port=CAN_0, CAN_Priority=3, S_overflow_flag=off, S_timestamp=off, sampletime=0.01}
      mask prompts: CAN_Port "CAN Port:"; CAN_Priority "Priority:"; S_overflow_flag "Send overflow flag"; S_timestamp "Send time stamp"
      mask init:
      | maskdisplay = cansendicon(CAN_Port,CAN_Priority,S_overflow_flag,S_timestamp);
      | set_param(gcb, 'MaskDisplay', maskdisplay);
      mask TypeOptions CAN_Port: CAN_0 | CAN_1 | CAN_2 | CAN_3
      mask TypeOptions CAN_Priority: 0 | 1 | 2 | 3 | 4 | 5 | 6 | 7
      mask Display: color('blue');text(0.98,0.9,'MPC5675K','horizontalAlignment','right');color('black');text(0.5,0.6,'FlexCAN_0 Send','horizontalAlignment','center');text(0.5,0.35,'Priority:3','horizontalAlignment','center');port_label('input',1,'CAN_Msg');
  CAN Send14 : S-Function  FunctionName=CAN_Send_P  Parameters=uint8(CAN_Port-1),uint8(CAN_Priority-1),uint8(S_overflow_flag),uint8(S_timestamp),double(sampletime)  SFunctionDeploymentMode=off  EnableBusSupport=off  mask{CAN_Port=CAN_0, CAN_Priority=3, S_overflow_flag=off, S_timestamp=off, sampletime=0.01}
      mask prompts: CAN_Port "CAN Port:"; CAN_Priority "Priority:"; S_overflow_flag "Send overflow flag"; S_timestamp "Send time stamp"
      mask init:
      | maskdisplay = cansendicon(CAN_Port,CAN_Priority,S_overflow_flag,S_timestamp);
      | set_param(gcb, 'MaskDisplay', maskdisplay);
      mask TypeOptions CAN_Port: CAN_0 | CAN_1 | CAN_2 | CAN_3
      mask TypeOptions CAN_Priority: 0 | 1 | 2 | 3 | 4 | 5 | 6 | 7
      mask Display: color('blue');text(0.98,0.9,'MPC5675K','horizontalAlignment','right');color('black');text(0.5,0.6,'FlexCAN_0 Send','horizontalAlignment','center');text(0.5,0.35,'Priority:3','horizontalAlignment','center');port_label('input',1,'CAN_Msg');
  CAN Send15 : S-Function  FunctionName=CAN_Send_P  Parameters=uint8(CAN_Port-1),uint8(CAN_Priority-1),uint8(S_overflow_flag),uint8(S_timestamp),double(sampletime)  SFunctionDeploymentMode=off  EnableBusSupport=off  mask{CAN_Port=CAN_0, CAN_Priority=3, S_overflow_flag=off, S_timestamp=off, sampletime=0.01}
      mask prompts: CAN_Port "CAN Port:"; CAN_Priority "Priority:"; S_overflow_flag "Send overflow flag"; S_timestamp "Send time stamp"
      mask init:
      | maskdisplay = cansendicon(CAN_Port,CAN_Priority,S_overflow_flag,S_timestamp);
      | set_param(gcb, 'MaskDisplay', maskdisplay);
      mask TypeOptions CAN_Port: CAN_0 | CAN_1 | CAN_2 | CAN_3
      mask TypeOptions CAN_Priority: 0 | 1 | 2 | 3 | 4 | 5 | 6 | 7
      mask Display: color('blue');text(0.98,0.9,'MPC5675K','horizontalAlignment','right');color('black');text(0.5,0.6,'FlexCAN_0 Send','horizontalAlignment','center');text(0.5,0.35,'Priority:3','horizontalAlignment','center');port_label('input',1,'CAN_Msg');
  CAN Send16 : S-Function  FunctionName=CAN_Send_P  Parameters=uint8(CAN_Port-1),uint8(CAN_Priority-1),uint8(S_overflow_flag),uint8(S_timestamp),double(sampletime)  SFunctionDeploymentMode=off  EnableBusSupport=off  mask{CAN_Port=CAN_0, CAN_Priority=3, S_overflow_flag=off, S_timestamp=off, sampletime=0.01}
      mask prompts: CAN_Port "CAN Port:"; CAN_Priority "Priority:"; S_overflow_flag "Send overflow flag"; S_timestamp "Send time stamp"
      mask init:
      | maskdisplay = cansendicon(CAN_Port,CAN_Priority,S_overflow_flag,S_timestamp);
      | set_param(gcb, 'MaskDisplay', maskdisplay);
      mask TypeOptions CAN_Port: CAN_0 | CAN_1 | CAN_2 | CAN_3
      mask TypeOptions CAN_Priority: 0 | 1 | 2 | 3 | 4 | 5 | 6 | 7
      mask Display: color('blue');text(0.98,0.9,'MPC5675K','horizontalAlignment','right');color('black');text(0.5,0.6,'FlexCAN_0 Send','horizontalAlignment','center');text(0.5,0.35,'Priority:3','horizontalAlignment','center');port_label('input',1,'CAN_Msg');
  CAN Send19 : S-Function  FunctionName=CAN_Send_P  Parameters=uint8(CAN_Port-1),uint8(CAN_Priority-1),uint8(S_overflow_flag),uint8(S_timestamp),double(sampletime)  SFunctionDeploymentMode=off  EnableBusSupport=off  mask{CAN_Port=CAN_0, CAN_Priority=3, S_overflow_flag=off, S_timestamp=off, sampletime=0.01}
      mask prompts: CAN_Port "CAN Port:"; CAN_Priority "Priority:"; S_overflow_flag "Send overflow flag"; S_timestamp "Send time stamp"
      mask init:
      | maskdisplay = cansendicon(CAN_Port,CAN_Priority,S_overflow_flag,S_timestamp);
      | set_param(gcb, 'MaskDisplay', maskdisplay);
      mask TypeOptions CAN_Port: CAN_0 | CAN_1 | CAN_2 | CAN_3
      mask TypeOptions CAN_Priority: 0 | 1 | 2 | 3 | 4 | 5 | 6 | 7
      mask Display: color('blue');text(0.98,0.9,'MPC5675K','horizontalAlignment','right');color('black');text(0.5,0.6,'FlexCAN_0 Send','horizontalAlignment','center');text(0.5,0.35,'Priority:3','horizontalAlignment','center');port_label('input',1,'CAN_Msg');
  CAN Send2 : S-Function  FunctionName=CAN_Send_P  Parameters=uint8(CAN_Port-1),uint8(CAN_Priority-1),uint8(S_overflow_flag),uint8(S_timestamp),double(sampletime)  SFunctionDeploymentMode=off  EnableBusSupport=off  mask{CAN_Port=CAN_0, CAN_Priority=3, S_overflow_flag=off, S_timestamp=off, sampletime=0.01}
      mask prompts: CAN_Port "CAN Port:"; CAN_Priority "Priority:"; S_overflow_flag "Send overflow flag"; S_timestamp "Send time stamp"
      mask init:
      | maskdisplay = cansendicon(CAN_Port,CAN_Priority,S_overflow_flag,S_timestamp);
      | set_param(gcb, 'MaskDisplay', maskdisplay);
      mask TypeOptions CAN_Port: CAN_0 | CAN_1 | CAN_2 | CAN_3
      mask TypeOptions CAN_Priority: 0 | 1 | 2 | 3 | 4 | 5 | 6 | 7
      mask Display: color('blue');text(0.98,0.9,'MPC5675K','horizontalAlignment','right');color('black');text(0.5,0.6,'FlexCAN_0 Send','horizontalAlignment','center');text(0.5,0.35,'Priority:3','horizontalAlignment','center');port_label('input',1,'CAN_Msg');
  CAN Send4 : S-Function  FunctionName=CAN_Send_P  Parameters=uint8(CAN_Port-1),uint8(CAN_Priority-1),uint8(S_overflow_flag),uint8(S_timestamp),double(sampletime)  SFunctionDeploymentMode=off  EnableBusSupport=off  mask{CAN_Port=CAN_0, CAN_Priority=3, S_overflow_flag=off, S_timestamp=off, sampletime=0.01}
      mask prompts: CAN_Port "CAN Port:"; CAN_Priority "Priority:"; S_overflow_flag "Send overflow flag"; S_timestamp "Send time stamp"
      mask init:
      | maskdisplay = cansendicon(CAN_Port,CAN_Priority,S_overflow_flag,S_timestamp);
      | set_param(gcb, 'MaskDisplay', maskdisplay);
      mask TypeOptions CAN_Port: CAN_0 | CAN_1 | CAN_2 | CAN_3
      mask TypeOptions CAN_Priority: 0 | 1 | 2 | 3 | 4 | 5 | 6 | 7
      mask Display: color('blue');text(0.98,0.9,'MPC5675K','horizontalAlignment','right');color('black');text(0.5,0.6,'FlexCAN_0 Send','horizontalAlignment','center');text(0.5,0.35,'Priority:3','horizontalAlignment','center');port_label('input',1,'CAN_Msg');
  CAN Send5 : S-Function  FunctionName=CAN_Send_P  Parameters=uint8(CAN_Port-1),uint8(CAN_Priority-1),uint8(S_overflow_flag),uint8(S_timestamp),double(sampletime)  SFunctionDeploymentMode=off  EnableBusSupport=off  mask{CAN_Port=CAN_0, CAN_Priority=3, S_overflow_flag=off, S_timestamp=off, sampletime=0.01}
      mask prompts: CAN_Port "CAN Port:"; CAN_Priority "Priority:"; S_overflow_flag "Send overflow flag"; S_timestamp "Send time stamp"
      mask init:
      | maskdisplay = cansendicon(CAN_Port,CAN_Priority,S_overflow_flag,S_timestamp);
      | set_param(gcb, 'MaskDisplay', maskdisplay);
      mask TypeOptions CAN_Port: CAN_0 | CAN_1 | CAN_2 | CAN_3
      mask TypeOptions CAN_Priority: 0 | 1 | 2 | 3 | 4 | 5 | 6 | 7
      mask Display: color('blue');text(0.98,0.9,'MPC5675K','horizontalAlignment','right');color('black');text(0.5,0.6,'FlexCAN_0 Send','horizontalAlignment','center');text(0.5,0.35,'Priority:3','horizontalAlignment','center');port_label('input',1,'CAN_Msg');
  CAN Send6 : S-Function  FunctionName=CAN_Send_P  Parameters=uint8(CAN_Port-1),uint8(CAN_Priority-1),uint8(S_overflow_flag),uint8(S_timestamp),double(sampletime)  SFunctionDeploymentMode=off  EnableBusSupport=off  mask{CAN_Port=CAN_0, CAN_Priority=3, S_overflow_flag=off, S_timestamp=off, sampletime=0.01}
      mask prompts: CAN_Port "CAN Port:"; CAN_Priority "Priority:"; S_overflow_flag "Send overflow flag"; S_timestamp "Send time stamp"
      mask init:
      | maskdisplay = cansendicon(CAN_Port,CAN_Priority,S_overflow_flag,S_timestamp);
      | set_param(gcb, 'MaskDisplay', maskdisplay);
      mask TypeOptions CAN_Port: CAN_0 | CAN_1 | CAN_2 | CAN_3
      mask TypeOptions CAN_Priority: 0 | 1 | 2 | 3 | 4 | 5 | 6 | 7
      mask Display: color('blue');text(0.98,0.9,'MPC5675K','horizontalAlignment','right');color('black');text(0.5,0.6,'FlexCAN_0 Send','horizontalAlignment','center');text(0.5,0.35,'Priority:3','horizontalAlignment','center');port_label('input',1,'CAN_Msg');
  CAN Send9 : S-Function  FunctionName=CAN_Send_P  Parameters=uint8(CAN_Port-1),uint8(CAN_Priority-1),uint8(S_overflow_flag),uint8(S_timestamp),double(sampletime)  SFunctionDeploymentMode=off  EnableBusSupport=off  mask{CAN_Port=CAN_0, CAN_Priority=3, S_overflow_flag=off, S_timestamp=off, sampletime=0.01}
      mask prompts: CAN_Port "CAN Port:"; CAN_Priority "Priority:"; S_overflow_flag "Send overflow flag"; S_timestamp "Send time stamp"
      mask init:
      | maskdisplay = cansendicon(CAN_Port,CAN_Priority,S_overflow_flag,S_timestamp);
      | set_param(gcb, 'MaskDisplay', maskdisplay);
      mask TypeOptions CAN_Port: CAN_0 | CAN_1 | CAN_2 | CAN_3
      mask TypeOptions CAN_Priority: 0 | 1 | 2 | 3 | 4 | 5 | 6 | 7
      mask Display: color('blue');text(0.98,0.9,'MPC5675K','horizontalAlignment','right');color('black');text(0.5,0.6,'FlexCAN_0 Send','horizontalAlignment','center');text(0.5,0.35,'Priority:3','horizontalAlignment','center');port_label('input',1,'CAN_Msg');
  Data Type Conversion{,1..10,19..24,29..41,46..61,70..105,107..109} (85 alike) : DataTypeConversion  OutDataTypeStr=single
  Gain1 : Gain  Gain=1000  OutDataTypeStr=Inherit: Same as input
  Gain{4,8,10,20,26,31,33,36} (8 alike) : Gain  Gain=10  OutDataTypeStr=Inherit: Same as input
  Gain13 : Gain  Gain=-1  OutDataTypeStr=single
  Gain{3,7,9,19,23..25,27,34..35} (10 alike) : Gain  Gain=180/pi  OutDataTypeStr=Inherit: Same as input
  Gain2 : Gain  Gain=1000  OutDataTypeStr=Inherit: Same as input
  wires:
  CAN Pack15/1 -> CAN Send2/1
  CAN Pack16/1 -> CAN Send15/1
  CAN Pack17/1 -> CAN Send16/1
  CAN Pack6/1 -> CAN Send14/1
  Bus Selector3/1 -> Gain13/1  "<DvtCalc_lLftDvt>"
  Bus Selector3/2 -> Data Type Conversion24/1  "<DvtCalc_lRgtDvt>"
  Data Type Conversion32/1 -> CAN Pack6/1
  Data Type Conversion1/1 -> CAN Pack6/2
  Data Type Conversion2/1 -> CAN Pack6/3
  Data Type Conversion21/1 -> CAN Pack17/1
  Data Type Conversion22/1 -> CAN Pack17/2
  Data Type Conversion23/1 -> CAN Pack17/3
  Data Type Conversion24/1 -> CAN Pack17/4
  [LMC_bsLLMon] -> Bus Selector3/1
  [LMC_bsLLMon] -> Bus Selector5/1
  [LMC_bsLLMon] -> Bus Selector6/1
  CAN Pack1/1 -> CAN Send1/1
  [LMC_bsLLMon] -> Bus Selector7/1
  Data Type Conversion34/1 -> CAN Pack15/1
  Data Type Conversion35/1 -> CAN Pack15/2
  Data Type Conversion36/1 -> CAN Pack15/3
  Data Type Conversion37/1 -> CAN Pack15/4
  Data Type Conversion29/1 -> CAN Pack16/1
  Data Type Conversion30/1 -> CAN Pack16/2
  Data Type Conversion31/1 -> CAN Pack16/3
  Data Type Conversion33/1 -> CAN Pack16/4
  Data Type Conversion38/1 -> CAN Pack1/1
  Data Type Conversion39/1 -> CAN Pack1/2
  Data Type Conversion40/1 -> CAN Pack1/3
  Data Type Conversion41/1 -> CAN Pack1/4
  Bus Selector5/2 -> Data Type Conversion35/1  "<RgtTTLC>"
  Bus Selector6/2 -> Data Type Conversion30/1  "<PrvwDvtRgt>"
  Bus Selector7/3 -> Gain1/1  "<PrvwCrvt_crPrvwCrvtLft>"
  Bus Selector7/4 -> Gain2/1  "<PrvwCrvt_crPrvwCrvtRgt>"
  CAN Pack3/1 -> CAN Send19/1
  Data Type Conversion/1 -> CAN Pack3/1
  Data Type Conversion46/1 -> CAN Pack3/2
  Data Type Conversion47/1 -> CAN Pack3/3
  Data Type Conversion48/1 -> CAN Pack3/4
  [LMC_bsLLMon] -> Bus Selector9/1
  Bus Selector9/3 -> Gain9/1  "<HdAgMax>"
  Bus Selector9/4 -> Gain7/1  "<SwtCon_bsSwtConMon>"
  Gain7/1 -> Gain8/1
  Gain8/1 -> Data Type Conversion48/1
  Gain9/1 -> Gain10/1
  Gain10/1 -> Data Type Conversion47/1
  CAN Pack4/1 -> CAN Send4/1
  Data Type Conversion52/1 -> CAN Pack4/4
  Data Type Conversion51/1 -> CAN Pack4/3
  Data Type Conversion50/1 -> CAN Pack4/2
  Data Type Conversion49/1 -> CAN Pack4/1
  [LMC_bsLLMon] -> Bus Selector10/1
  ? -> Data Type Conversion22/1  "<LKATG_lDesDvt>"
  ? -> Gain19/1  "<LKATG_phiDesHdAg>"
  Gain19/1 -> Gain20/1
  Gain20/1 -> Data Type Conversion21/1
  Bus Selector7/1 -> Gain35/1  "<PrdcHdAgLft_phiPrvwHdAgLft>"
  Bus Selector7/2 -> Gain34/1  "<PrdcHdAgRgt_phiPrvwHdAgRgt>"
  Bus Selector6/3 -> Gain25/1  "<PrdcHdAgLft_phiPrdcHdAgLft>"
  Bus Selector6/4 -> Gain27/1  "<PrdcHdAgRgt_phiPrdcHdAgRgt>"
  Gain13/1 -> Data Type Conversion23/1
  CAN Pack5/1 -> CAN Send5/1
  CAN Pack7/1 -> CAN Send6/1
  [LMC_bsLLMon] -> Bus Selector11/1
  Data Type Conversion54/1 -> CAN Pack7/1
  Bus Selector11/2 -> Data Type Conversion55/1  "<LKAPhSM_stLKAPhFlg>"
  Data Type Conversion55/1 -> CAN Pack7/2
  Bus Selector11/3 -> Data Type Conversion56/1  "<ExFlg>"
  Data Type Conversion56/1 -> CAN Pack7/3
  Data Type Conversion61/1 -> CAN Pack7/4
  Bus Selector11/4 -> Data Type Conversion61/1  "<SwtConFlg>"
  Bus Selector11/1 -> Data Type Conversion54/1  "<ToDeactvCFlg>"
  Bus Selector9/1 -> Gain23/1  "<UndrLim_phiSWAMax>"
  Gain23/1 -> Data Type Conversion/1
  Bus Selector9/2 -> Gain24/1  "<UndrLim_dphiSWARMax>"
  Gain24/1 -> Data Type Conversion46/1
  Bus Selector5/1 -> Data Type Conversion34/1  "<LftTTLC>"
  Bus Selector6/1 -> Data Type Conversion29/1  "<PrvwDvtLft>"
  CAN Pack10/1 -> CAN Send9/1
  Data Type Conversion72/1 -> CAN Pack10/3
  Data Type Conversion70/1 -> CAN Pack10/1
  Data Type Conversion71/1 -> CAN Pack10/2
  Data Type Conversion73/1 -> CAN Pack10/4
  Gain31/1 -> Data Type Conversion39/1
  Gain34/1 -> Gain31/1
  Gain35/1 -> Gain36/1
  Gain36/1 -> Data Type Conversion38/1
  Bus Selector5/3 -> Data Type Conversion36/1  "<PrdcDvt_lPrdcDvtLft>"
  Bus Selector5/4 -> Data Type Conversion37/1  "<PrdcDvt_lPrdcDvtRgt>"
  Gain25/1 -> Gain26/1
  Gain26/1 -> Data Type Conversion31/1
  Gain27/1 -> Gain33/1
  Gain33/1 -> Data Type Conversion33/1
  Gain1/1 -> Data Type Conversion40/1
  Gain2/1 -> Data Type Conversion41/1
  Bus Selector10/1 -> Data Type Conversion49/1  "<phiSWACmd>"
  Bus Selector10/2 -> Data Type Conversion50/1  "<PrdcDvt_lPrdcDvt>"
  Bus Selector10/3 -> Gain3/1  "<PrdcHdAg_phiPrdcHdAg>"
  Gain3/1 -> Gain4/1
  Gain4/1 -> Data Type Conversion51/1
  [LMC_bsLLMon] -> Bus Selector1/1
  [LL_bsInInfoSyn] -> Bus Selector/1
  Bus Selector/1 -> Data Type Conversion32/1  "<EPSRx_stEPSCtlState>"
  Bus Selector1/1 -> Data Type Conversion1/1  "<LKA_State>"
  Bus Selector1/2 -> Data Type Conversion2/1  "<LDW_State>"
  [LL_bsInInfoSyn] -> Bus Selector2/1
  Bus Selector2/1 -> Data Type Conversion19/1  "<SWARx_phiSWA>"
  [LMC_bsLLMon] -> Bus Selector12/1
  Bus Selector12/1 -> Data Type Conversion20/1  "<DvtCalc_lLftDvt>"
  Bus Selector12/2 -> Data Type Conversion53/1  "<DvtCalc_lRgtDvt>"
  [LL_bsInInfoSyn] -> Bus Selector15/1
  Bus Selector15/1 -> Data Type Conversion75/1  "<CmrRxPrcs_facmL0C0>"
  Bus Selector15/2 -> Data Type Conversion76/1  "<CmrRxPrcs_facmR0C0>"
  Data Type Conversion74/1 -> CAN Pack11/1
  Data Type Conversion19/1 -> CAN Pack11/3
  Data Type Conversion20/1 -> CAN Pack12/1
  Data Type Conversion53/1 -> CAN Pack12/2
  Data Type Conversion75/1 -> CAN Pack12/3
  Data Type Conversion76/1 -> CAN Pack12/4
  CAN Pack11/1 -> CAN Send10/1
  CAN Pack12/1 -> CAN Send11/1
  [LKA_CAL_SWA_CMD] -> Data Type Conversion74/1
  [LKA_SWA_CMD] -> CAN Pack11/2
  Data Type Conversion84/1 -> CAN Pack5/20  "ob_LKA_Deactive_EPS"
  Data Type Conversion80/1 -> CAN Pack5/16  "ob_LKA_Active_ThresActvFlg"
  Data Type Conversion79/1 -> CAN Pack5/15  "ob_LKA_Active_EPS"
  Bus Selector18/6 -> Data Type Conversion77/1  "<DISABLE_LDWALRMT>"
  Bus Selector18/5 -> Data Type Conversion10/1  "<LKAOWN>"
  Bus Selector18/4 -> Data Type Conversion9/1  "<DRIVER>"
  Data Type Conversion8/1 -> CAN Pack5/10  "ob_LKA_Disable_Lane"
  Data Type Conversion77/1 -> CAN Pack5/13  "ob_LKA_Disable_LDWAlrmt"
  Bus Selector18/3 -> Data Type Conversion8/1  "<LANE>"
  [LMC_bsLLMon] -> Bus Selector18/1
  Data Type Conversion10/1 -> CAN Pack5/12  "ob_LKA_Disable_LKAOwn"
  Data Type Conversion7/1 -> CAN Pack5/9  "ob_LKA_Disable_VehState"
  Data Type Conversion6/1 -> CAN Pack5/8  "ob_LKA_Disable_Disable"
  Bus Selector17/7 -> Data Type Conversion5/1  "<LKAOWN>"
  Bus Selector17/3 -> Data Type Conversion58/1  "<VEHSTATE>"
  Bus Selector17/2 -> Data Type Conversion57/1  "<ENA_DACMODE>"
  Data Type Conversion59/1 -> CAN Pack5/4  "ob_LKA_Enable_Lane"
  Data Type Conversion57/1 -> CAN Pack5/2  "ob_LKA_Enable_DACMode"
  Data Type Conversion3/1 -> CAN Pack5/1  "ob_LKA_Enable_Enable"
  Bus Selector17/1 -> Data Type Conversion3/1  "<ENA_ENA>"
  Data Type Conversion85/1 -> CAN Pack5/21  "ob_LKA_Deactive_ToDeactive"
  Data Type Conversion94/1 -> CAN Pack13/9  "ob_LKA_Enable_LKAOwn_EPS"
  Data Type Conversion78/1 -> CAN Pack5/14  "ob_LKA_Active_Active"
  Data Type Conversion99/1 -> CAN Pack13/14  "ob_LKA_Disable_VehState_LIGHT"
  Data Type Conversion108/1 -> CAN Pack13/22  "ob_LKA_Disable_LKAOwn_VehPos"
  Data Type Conversion103/1 -> CAN Pack13/18  "ob_LKA_Disable_Lane_Curvate"
  Data Type Conversion101/1 -> CAN Pack13/16  "ob_LKA_Disable_Lane_Quality"
  Data Type Conversion90/1 -> CAN Pack13/5  "ob_LKA_Enable_Lane_Width"
  Bus Selector20/11 -> Data Type Conversion96/1  "<LKAOWN_VEHPOS>"
  Bus Selector17/4 -> Data Type Conversion59/1  "<LANE>"
  [LMC_bsLLMon] -> Bus Selector21/1
  Bus Selector19/1 -> Data Type Conversion78/1  "<ACTIVE>"
  Bus Selector20/9 -> Data Type Conversion94/1  "<LKAOWN_EPS>"
  Bus Selector19/5 -> Data Type Conversion82/1  "<DEACTIVE>"
  Data Type Conversion98/1 -> CAN Pack13/13  "ob_LKA_Disable_VehState_VehSpd"
  Data Type Conversion89/1 -> CAN Pack13/4  "ob_LKA_Enable_Lane_Quality"
  Bus Selector20/7 -> Data Type Conversion92/1  "<DRIVERINT_ACTION>"
  Data Type Conversion9/1 -> CAN Pack5/11  "ob_LKA_Disable_DriverInt"
  Bus Selector17/6 -> Data Type Conversion4/1  "<ENA_LDWOWN>"
  Data Type Conversion100/1 -> CAN Pack13/15  "ob_LKA_Disable_VehState_Gear"
  Bus Selector20/3 -> Data Type Conversion88/1  "<VEHSTATE_GEAR>"
  Data Type Conversion88/1 -> CAN Pack13/3  "ob_LKA_Enable_VehState_Gear"
  Data Type Conversion87/1 -> CAN Pack13/2  "ob_LKA_Enable_VehState_LIGHT"
  Data Type Conversion58/1 -> CAN Pack5/3  "ob_LKA_Enable_VehState"
  Bus Selector21/1 -> Data Type Conversion98/1  "<VEHSTATE_SPEED>"
  Bus Selector20/2 -> Data Type Conversion87/1  "<VEHSTATE_LIGHT>"
  Bus Selector19/4 -> Data Type Conversion81/1  "<ACTIVE_LANEQUALITY>"
  Bus Selector20/5 -> Data Type Conversion90/1  "<LANE_WIDTH>"
  Data Type Conversion109/1 -> CAN Pack13/23  "ob_LKA_Disable_LKAOwn_EPS"
  Bus Selector18/1 -> Data Type Conversion6/1  "<DISABLE>"
  Bus Selector21/11 -> Data Type Conversion109/1  "<LKAOWN_EPS>"
  Data Type Conversion60/1 -> CAN Pack5/5  "ob_LKA_Enable_DriverInt"
  [LMC_bsLLMon] -> Bus Selector17/1
  Data Type Conversion92/1 -> CAN Pack13/7  "ob_LKA_Enable_DriverInt_Action"
  Data Type Conversion91/1 -> CAN Pack13/6  "ob_LKA_Enable_Lane_Curvate"
  Data Type Conversion4/1 -> CAN Pack5/6  "ob_LKA_Enable_LDWOwn"
  Bus Selector21/9 -> Data Type Conversion107/1  "<LKAOWN_VEHLATSPEED>"
  Bus Selector20/4 -> Data Type Conversion89/1  "<LANE_QUALITY>"
  Bus Selector21/7 -> Data Type Conversion104/1  "<DRIVER_ACT>"
  Data Type Conversion86/1 -> CAN Pack13/1  "ob_LKA_Enable_VehState_VehSpd"
  Bus Selector19/8 -> Data Type Conversion85/1  "<DEACTIVE_TODEACTIVE>"
  Bus Selector20/8 -> Data Type Conversion93/1  "<DRIVERINT_RELEASE>"
  Bus Selector21/8 -> Data Type Conversion105/1  "<DRIVER_RELEASE>"
  Bus Selector19/2 -> Data Type Conversion79/1  "<ACTIVE_EPS>"
  Bus Selector20/1 -> Data Type Conversion86/1  "<VEHSTATE_VEHSPEED>"
  [LMC_bsLLMon] -> Bus Selector20/1
  Data Type Conversion83/1 -> CAN Pack5/19  "ob_LKA_Deactive_Thres"
  Data Type Conversion104/1 -> CAN Pack13/19  "ob_LKA_Disable_DriverInt_Action"
  Bus Selector21/2 -> Data Type Conversion99/1  "<VEHSTATE_LIGHT>"
  Bus Selector19/6 -> Data Type Conversion83/1  "<DEACTIVE_THRES>"
  Bus Selector19/7 -> Data Type Conversion84/1  "<DEACTIVE_EPS>"
  Data Type Conversion5/1 -> CAN Pack5/7  "ob_LKA_Enable_LKAOwn"
  Bus Selector18/2 -> Data Type Conversion7/1  "<VEHSTATE>"
  Bus Selector19/3 -> Data Type Conversion80/1  "<DvtThresActvFlg>"
  Bus Selector21/5 -> Data Type Conversion102/1  "<LANE_WIDTH>"
  Data Type Conversion82/1 -> CAN Pack5/18  "ob_LKA_Deactive_Deactive"
  Data Type Conversion81/1 -> CAN Pack5/17  "ob_LKA_Active_LaneQuality"
  [LMC_bsLLMon] -> Bus Selector19/1
  Bus Selector20/6 -> Data Type Conversion91/1  "<LANE_CURVAT>"
  Data Type Conversion105/1 -> CAN Pack13/20  "ob_LKA_Disable_DriverInt_Release"
  Bus Selector21/4 -> Data Type Conversion101/1  "<LANE_QUALITY>"
  Bus Selector20/10 -> Data Type Conversion95/1  "<LKAOWN_VEHLSPD>"
  Bus Selector21/3 -> Data Type Conversion100/1  "<VEHSTATE_GEAR>"
  Data Type Conversion102/1 -> CAN Pack13/17  "ob_LKA_Disable_Lane_Width"
  Data Type Conversion96/1 -> CAN Pack13/11  "ob_LKA_Enable_LKAOwn_VehPos"
  Bus Selector21/6 -> Data Type Conversion103/1  "<LANE_CURVAT>"
  Data Type Conversion97/1 -> CAN Pack13/12  "ob_LKA_Enable_LKAOwn_ExitLane"
  Data Type Conversion107/1 -> CAN Pack13/21  "ob_LKA_Disable_LKAOwn_VehLatSpd"
  Bus Selector20/12 -> Data Type Conversion97/1  "<LKAOWN_EXITLANE>"
  Bus Selector17/5 -> Data Type Conversion60/1  "<DRIVERINT>"
  Data Type Conversion95/1 -> CAN Pack13/10  "ob_LKA_Enable_LKAOwn_VehLatSpd"
  Bus Selector21/10 -> Data Type Conversion108/1  "<LKAOWN_VEHPOS>"
  Data Type Conversion93/1 -> CAN Pack13/8  "ob_LKA_Enable_DriverInt_Release"
  CAN Pack13/1 -> CAN Send12/1
